simulink model "MainDriveV1"  (Simulink 7.6)
settings: Solver=ode45  StartTime=0.0  StopTime=SimulTime  RelTol=1e-3
values from neighbouring files (symbols this model uses):
  R = 25    [ParamtersSpindel.m]    (also in PlottingSpindel.m = Scp_MainDriveT.signals(3).values(:,1)/1000; PlottingSpindel_Kuehlung.m = Scp_MainDriveT.signals(3).values(:,1)/1000)
  sb = 5.67*(10^-8)    (= 5.67e-08)    [ParamtersSpindel.m]
  T_amb = 295    [ParamtersSpindel.m]
undefined symbols (not defined in the file or in its folder): magnitude, MainDrive
settings Model: Creator=Coni  LastModifiedBy=conid

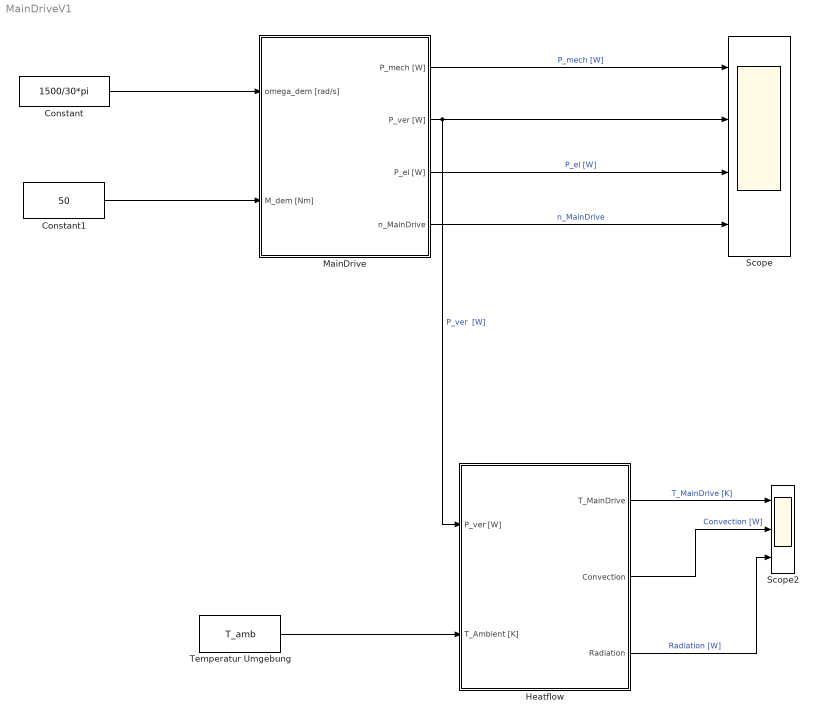
== system MainDriveV1 ==
  Constant : Constant  Value=1500/30*pi
  Constant1 : Constant  Value=50
  Heatflow : Subsystem  TreatAsAtomicUnit=on
  MainDrive : Subsystem  TreatAsAtomicUnit=on
  Scope : Scope  NumInputPorts=4
      settings: TickLabels=on  TimeRange=100  YMin=0~-5000~-2000~-0.1  YMax=16000~30000~14000~0.9  SaveName=Scp_MainDrive
  Scope2 : Scope  NumInputPorts=3
      settings: TickLabels=on  YMin=281.2~-1e-012~0  YMax=310.8~0~250  SaveName=Scp_MainDriveT
  Temperatur Umgebung : Constant  Value=T_amb
  wires:
  Constant/1 -> MainDrive/1(omega_dem [rad/s])
  Constant1/1 -> MainDrive/2(M_dem [Nm])
  MainDrive/1(P_mech [W]) -> Scope/1  "P_mech [W]"
  MainDrive/2(P_ver [W]) -> Heatflow/1(P_ver [W]), Scope/2  "P_ver  [W]"
  MainDrive/4(n_MainDrive) -> Scope/4  "n_MainDrive"
  Temperatur Umgebung/1 -> Heatflow/2(T_Ambient [K])
  Heatflow/1(T_MainDrive) -> Scope2/1  "T_MainDrive [K]"
  Heatflow/2(Convection) -> Scope2/2  "Convection [W]"
  Heatflow/3(Radiation) -> Scope2/3  "Radiation [W]"
  MainDrive/3(P_el [W]) -> Scope/3  "P_el [W]"

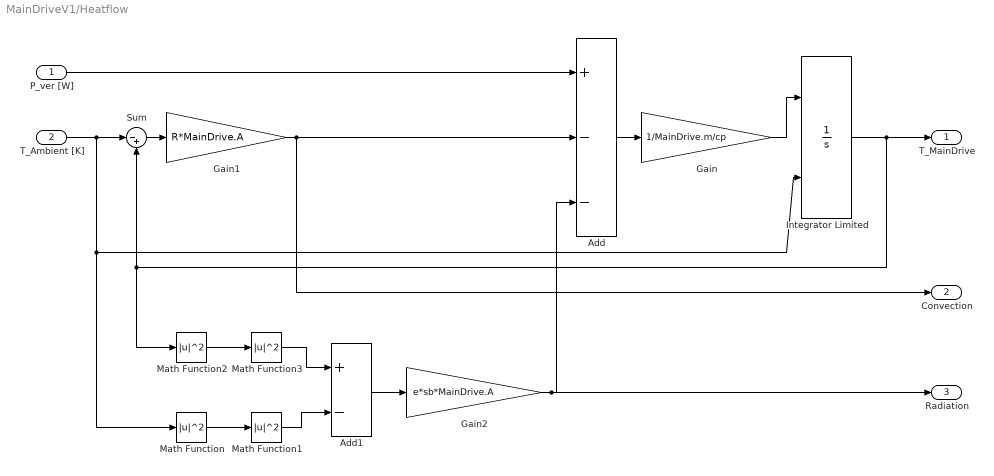
== system MainDriveV1/Heatflow ==
  P_ver [W] : Inport
  T_Ambient [K] : Inport  Port=2
  Add : Sum  Inputs=+--
  Add1 : Sum  Inputs=+-
  Gain : Gain  Gain=1/MainDrive.m/cp
  Gain1 : Gain  Gain=R*MainDrive.A
  Gain2 : Gain  Gain=e*sb*MainDrive.A
  Integrator Limited : Integrator  InitialConditionSource=external  LimitOutput=on
  Math Function{,1..3} (4 alike) : Math  Operator=magnitude^2  SaturateOnIntegerOverflow=on
  Sum : Sum  Inputs=|-+
  T_MainDrive : Outport
  Convection : Outport  Port=2
  Radiation : Outport  Port=3
  wires:
  P_ver [W]/1 -> Add/1
  T_Ambient [K]/1 -> Sum/1, Integrator Limited/2, Math Function/1
  Sum/1 -> Gain1/1
  Gain/1 -> Integrator Limited/1
  Gain1/1 -> Add/2, Convection/1
  Integrator Limited/1 -> T_MainDrive/1, Sum/2, Math Function2/1
  Add/1 -> Gain/1
  Math Function/1 -> Math Function1/1
  Gain2/1 -> Radiation/1, Add/3
  Math Function2/1 -> Math Function3/1
  Math Function1/1 -> Add1/2
  Math Function3/1 -> Add1/1
  Add1/1 -> Gain2/1

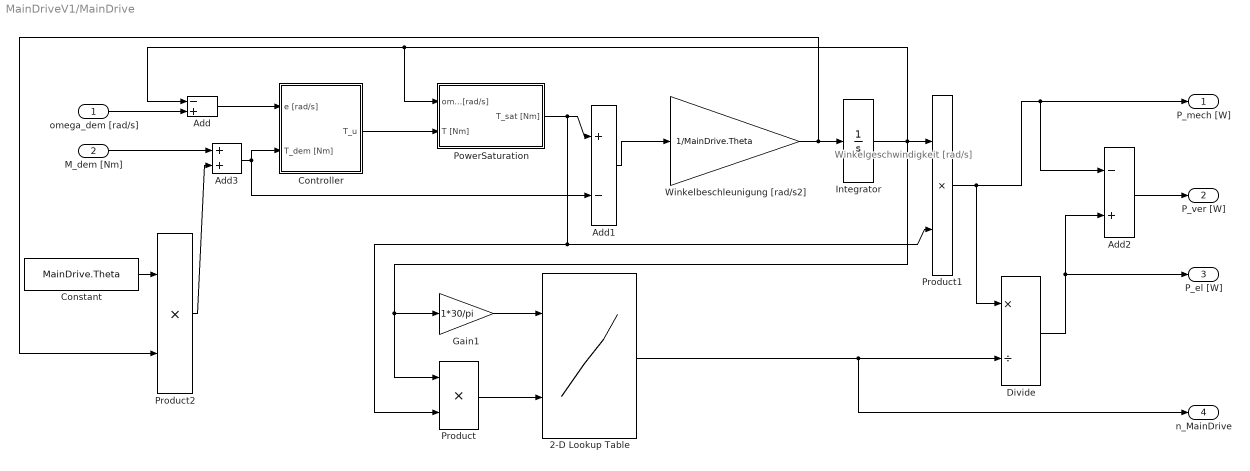
== system MainDriveV1/MainDrive ==
  note: Winkelgeschwindigkeit [rad/s]
  omega_dem [rad/s] : Inport
  M_dem [Nm] : Inport  Port=2
  2-D Lookup Table : Lookup_n-D  BreakpointsForDimension1=MainDrive.Tabelomega  BreakpointsForDimension2=MainDrive.TabelM  Table=MainDrive.Tabeleta  InterpMethod=Cubic spline  ExtrapMethod=Cubic spline  RndMeth=Simplest  InputSameDT=on
  Add : Sum  Inputs=-+
  Add1 : Sum  Inputs=+-
  Add2 : Sum  Inputs=-+
  Add3 : Sum
  Constant : Constant  Value=MainDrive.Theta
  Controller : Subsystem  TreatAsAtomicUnit=on
  Divide : Product  Inputs=*/
  Gain1 : Gain  Gain=1*30/pi
  Integrator : Integrator
  PowerSaturation : Subsystem  TreatAsAtomicUnit=on
  Product : Product  RndMeth=Zero
  Product1 : Product  RndMeth=Zero
  Product2 : Product  RndMeth=Zero
  Winkelbeschleunigung [rad/s2] : Gain  Gain=1/MainDrive.Theta
  P_mech [W] : Outport
  P_ver [W] : Outport  Port=2
  P_el [W] : Outport  Port=3
  n_MainDrive : Outport  Port=4
  wires:
  omega_dem [rad/s]/1 -> Add/2
  Add/1 -> Controller/1(e [rad/s])
  Controller/1(T_u) -> PowerSaturation/2(T [Nm])
  PowerSaturation/1(T_sat [Nm]) -> Add1/1, Product1/2, Product/2
  Add1/1 -> Winkelbeschleunigung [rad/s2]/1
  Winkelbeschleunigung [rad/s2]/1 -> Integrator/1, Product2/2
  Integrator/1 -> Product1/1, Add/1, PowerSaturation/1(omega [rad/s]), Product/1, Gain1/1
  Product1/1 -> Divide/1, P_mech [W]/1, Add2/1
  Add2/1 -> P_ver [W]/1
  Divide/1 -> Add2/2, P_el [W]/1
  2-D Lookup Table/1 -> Divide/2, n_MainDrive/1
  Product/1 -> 2-D Lookup Table/2
  Gain1/1 -> 2-D Lookup Table/1
  Constant/1 -> Product2/1
  Add3/1 -> Controller/2(T_dem [Nm]), Add1/2
  M_dem [Nm]/1 -> Add3/1
  Product2/1 -> Add3/2

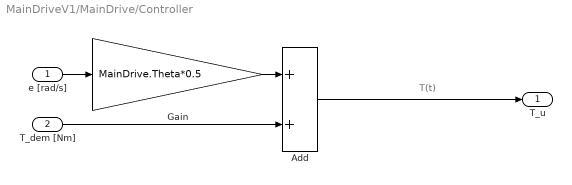
== system MainDriveV1/MainDrive/Controller ==
  note: T(t)
  e [rad/s] : Inport
  T_dem [Nm] : Inport  Port=2
  Add : Sum
  Gain : Gain  Gain=MainDrive.Theta*0.5
  T_u : Outport
  wires:
  Add/1 -> T_u/1
  T_dem [Nm]/1 -> Add/2
  Gain/1 -> Add/1
  e [rad/s]/1 -> Gain/1

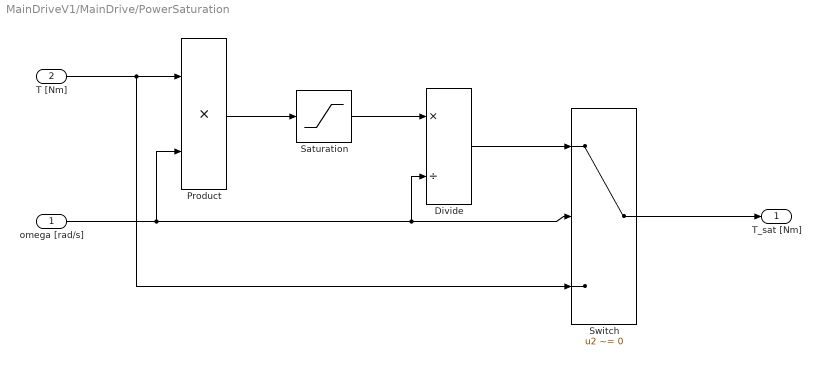
== system MainDriveV1/MainDrive/PowerSaturation ==
  omega [rad/s] : Inport
  T [Nm] : Inport  Port=2
  Divide : Product  Inputs=*/
  Product : Product  RndMeth=Zero
  Saturation : Saturate  UpperLimit=MainDrive.Pmax  LowerLimit=-MainDrive.Pmax
  Switch : Switch  Criteria=u2 ~= 0
  T_sat [Nm] : Outport
  wires:
  Product/1 -> Saturation/1
  Saturation/1 -> Divide/1
  Divide/1 -> Switch/1
  Switch/1 -> T_sat [Nm]/1
  T [Nm]/1 -> Product/1, Switch/3
  omega [rad/s]/1 -> Switch/2, Divide/2, Product/2
